simulink model "sf_custom"  (Simulink 7.6)
settings: Solver=ode3  StartTime=0.0  StopTime=20  MaxStep=.1  RelTol=1e-3
settings Model: Creator=The MathWorks Inc.  CovMetricSettings=dcmtr  ExtModeAutoUpdateStatusClock=off
settings DataIOCC: SignalLoggingName=sigsOut
settings OptimizationCC: BooleanDataType=off  InitFltsAndDblsToZero=on  OptimizeModelRefInitCode=on  LifeSpan=1  BufferReusableBoundary=off
settings DebuggingCC: CheckExecutionContextPreStartOutputMsg=on  CheckExecutionContextRuntimeOutputMsg=on  SignalResolutionControl=TryResolveAllWithWarning  SolverPrmCheckMsg=none  MultiTaskDSMMsg=warning  MultiTaskCondExecSysMsg=none  BusObjectLabelMismatch=none  StrictBusMsg=None
settings HardwareCC: TargetHWDeviceType=32-bit Generic
settings SFSimCC: SimCustomHeaderCode="#include \"my_header.h\""  SimUserSources=my_function.c  SimParseCustomCode=off
settings RTWCC: SystemTargetFile=ert.tlc  TemplateMakefile=ert_default_tmf  Description=RTW Embedded Coder (no auto configuration)  ProcessScript=ert_make_rtw_hook  CustomHeaderCode="#include \"my_header.h\""  CustomSource=my_function.c  IncludeERTFirstTime=on
settings CodeAppCC: IgnoreCustomStorageClasses=off
settings ERTTargetCC: MultiwordLength=2048  GenerateSampleERTMain=on  SupportContinuousTime=on  SupportNonInlinedSFcns=on  ERTCustomFileTemplate=example_file_process.tlc  ConvertIfToSwitch=off

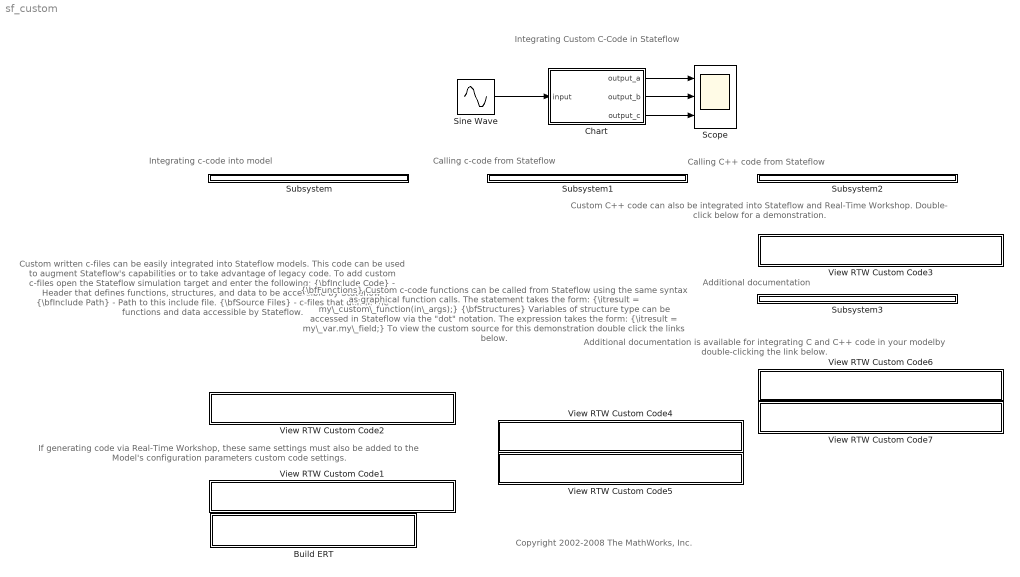
== system sf_custom ==
  note: Integrating Custom C-Code in Stateflow
  note: Calling C++ code from Stateflow
  note: Integrating c-code into model
  note: Calling c-code from Stateflow
  note: Custom written c-files can be easily integrated into
      | Stateflow models.  This code can be used to
      | augment Stateflow's capabilities or to take
      | advantage of legacy code.
      |
      | To add custom c-files open the Stateflow
      | simulation target and enter the following:
      |
      |   {\bfInclude Code} - Header that defines functions,
      |                               structures, and data to be
      |                               accessible by Stateflow.
      |   {\bfInclude Path} - Path to this include file.
      |   {\bfSource Files} - c-files that define the functions
      |                              and data accessible by Stateflow.
  note: If generating code via Real-Time Workshop, these
      | same settings must also be added to the Model's
      | configuration parameters custom code settings.
  note: {\bfFunctions}
      | Custom c-code functions can be called from
      | Stateflow using the same syntax as graphical
      | function calls.  The statement takes the form:
      |
      |   {\itresult = my\_custom\_function(in\_args);}
      |
      | {\bfStructures}
      | Variables of structure type can be accessed in
      | Stateflow via the "dot" notation.  The expression
      | takes the form:
      |
      |   {\itresult = my\_var.my\_field;}
      |
      | To view the custom source for this demonstration
      | double click the links below.
  note: Custom C++ code can also be integrated into
      | Stateflow and Real-Time Workshop.  Double-
      | click below for a demonstration.
  note: Additional documentation
  note: Additional documentation is available
      | for integrating C and C++ code in
      | your modelby double-clicking the link
      | below.
  note: Copyright 2002-2008 The MathWorks, Inc.
  Build ERT : Subsystem  mask{attrib_overrides={}}
      mask prompts: attrib_overrides "List of attributes to preserve (cell of strings):"
      mask help: Enter the attributes of the configuration set that you want preserved. Otherwise, the default configuration script will override your current settings.
      mask init:
      | pos    = get_param(gcb, 'Position');
      | width  = pos(3) - pos(1);
      | height = pos(4) - pos(2);
      | 
      | 
      | % Compute arrow coordinates
      | arrowW = width  / 20;
      | arrowH = height / 2.5;
      | arrowX = width  / 50;
      | arrowY = height / 3;
      | arrowXvec = [arrowX, arrowX, arrowX + arrowW];
      | arrowYvec = [arrowY, arrowY + arrowH, arrowY + arrowH / 2];
      | 
      | % Compute text position
      | textXbuff = width / 30;
      | textX  = arrowX + arrowW + textXbuff;
      | textY  = height / 2;
      settings: OpenFcn=|
      | model=bdroot;
      | rtwbuilddemomodel(model);
      mask Display:
      | patch(arrowXvec, arrowYvec);
      | text(textX, textY, 'Build model using Real-Time\nWorkshop');
  Chart : Stateflow chart  TreatAsAtomicUnit=on
  Scope : Scope  NumInputPorts=3
      settings: TimeRange=20  YMin=-4~-2~1  YMax=4~2~3.5
  Sine Wave : Sin  SampleTime=0
  Subsystem : Subsystem
  Subsystem1 : Subsystem
  Subsystem2 : Subsystem
  Subsystem3 : Subsystem
  View RTW Custom Code1 : Subsystem
      mask init: same as sf_custom/Build ERT
      settings: OpenFcn=|
      | slCfgPrmDlg(bdroot,'Open');
      | slCfgPrmDlg(bdroot,'TurnToPage','Real-Time Workshop/Custom Code');
      mask Display:
      | patch(arrowXvec, arrowYvec);
      | text(textX, textY, 'Open Real-Time Workshop\ncustom code settings');
  View RTW Custom Code2 : Subsystem
      mask init: same as sf_custom/Build ERT
      settings: OpenFcn=|
      | model = bdroot;
      | slCfgPrmDlg(model,'Open');
      | slCfgPrmDlg(bdroot,'TurnToPage','Simulation Target/Custom Code');
      | clear model;
      mask Display:
      | patch(arrowXvec, arrowYvec);
      | text(textX, textY, 'Open Stateflow simulation\ncustom code settings');
  View RTW Custom Code3 : Subsystem
      mask init: same as sf_custom/Build ERT
      settings: OpenFcn=sf_cpp
      mask Display:
      | patch(arrowXvec, arrowYvec);
      | text(textX, textY, 'Open sf_cpp');
  View RTW Custom Code4 : Subsystem
      mask init: same as sf_custom/Build ERT
      settings: OpenFcn=eval('edit my_header.h')
      mask Display:
      | patch(arrowXvec, arrowYvec);
      | text(textX, textY, 'Open my_header.h');
  View RTW Custom Code5 : Subsystem
      mask init: same as sf_custom/Build ERT
      settings: OpenFcn=eval('edit my_function.c')
      mask Display:
      | patch(arrowXvec, arrowYvec);
      | text(textX, textY, 'Open my_function.c');
  View RTW Custom Code6 : Subsystem
      mask init: same as sf_custom/Build ERT
      settings: OpenFcn=helpview([docroot '/mapfiles/stateflow.map'], 'TARGET_OPTIONS_DIALOG')
      mask Display:
      | patch(arrowXvec, arrowYvec);
      | text(textX, textY, 'C-Code integration');
  View RTW Custom Code7 : Subsystem
      mask init: same as sf_custom/Build ERT
      settings: OpenFcn=helpview([docroot '/mapfiles/stateflow.map'], 'including_custom_cpp_code')
      mask Display:
      | patch(arrowXvec, arrowYvec);
      | text(textX, textY, 'C++-Code integration');
  wires:
  Sine Wave/1 -> Chart/1(input)
  Chart/1(output_a) -> Scope/1
  Chart/2(output_b) -> Scope/2
  Chart/3(output_c) -> Scope/3

== system sf_custom/Build ERT ==

== system sf_custom/Subsystem ==

== system sf_custom/Subsystem1 ==

== system sf_custom/Subsystem2 ==

== system sf_custom/Subsystem3 ==

== system sf_custom/View RTW Custom Code1 ==

== system sf_custom/View RTW Custom Code2 ==

== system sf_custom/View RTW Custom Code3 ==

== system sf_custom/View RTW Custom Code4 ==

== system sf_custom/View RTW Custom Code5 ==

== system sf_custom/View RTW Custom Code6 ==

== system sf_custom/View RTW Custom Code7 ==

== stateflow chart Chart ==
  state One [parallel]
    settings: executionOrder=1
    state A
      during:
      gMyStructVar.a = input;
      output_a=gMyStructVar.a*3;
      output_b = my_function(input);
    (default) -> A
  state Two [parallel]
    settings: executionOrder=2
    state B
      during:
      gMyStructVar.b[1]=input+3;
      gMyStructPointerVar = &gMyStructVar;
      output_c=gMyStructPointerVar->b[1];
    (default) -> B
  note: In this demo, a C-code function defined in my_function.c and a structure that is defined
      | in my_header.h are included in the chart. MY_FUNCTION simply multiplies its input by
      | 2. The structure in my_header.h is defined as follows:
      | typedef struct {
      |                 real_T a;
      |                 int8_T b[10];
      | }MyStruct;
      | In the model, we access the structure member using the dot notation:  MyStruct.a and
      | also with the use of a pointer: gMyStructPointerVar ->b[1].  Notice that 'b' is defined as
      | an 8-bit integer value and not a Real (double) value. This the reason why 'output_c'
      | alternates between values '1' and '0' instead of taking the precise values of the input
      | sine wave.
  data: input input double; output_a output double; output_b output double; output_c output double
